simulink model "Lessons_Scheduled_Completed"  (R2024b)
settings: Solver=VariableStepAuto  StartTime=0.0  StopTime=365  RelTol=1e-3
undefined symbols (not defined in the file): m, n
settings Model: Creator=lerat  LastModifiedBy=lerat

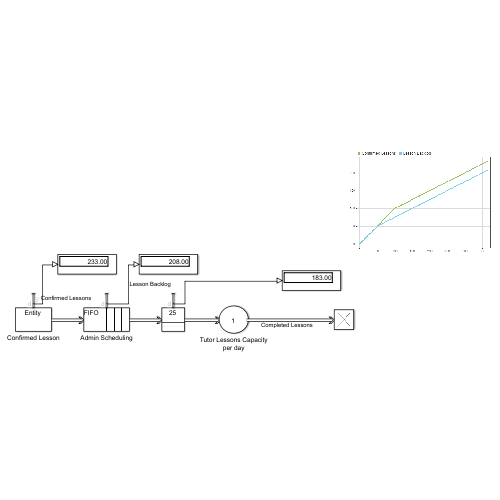
[thumbnail: Simulink's stored preview of the top-level diagram]
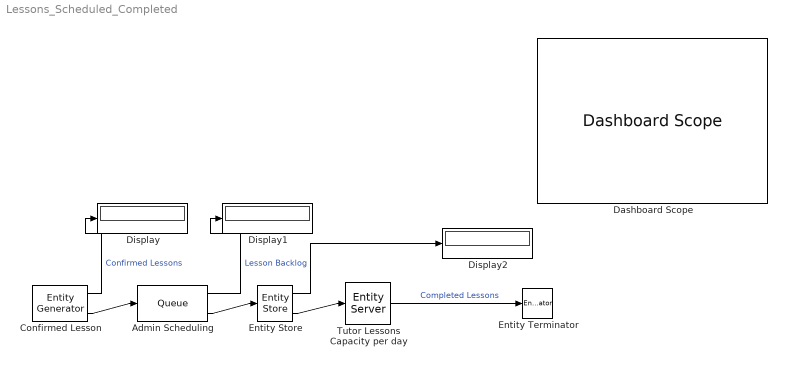
== system Lessons_Scheduled_Completed ==
  Admin Scheduling : Queue  InputPortMessageModes=m  OutputPortMessageModes=n,m  NumberEntitiesDeparted=on
      settings: OutputPortMap=o0,o5
  Confirmed Lesson : EntityGenerator  OutputPortMessageModes=n,m  NumberEntitiesDeparted=on  EntityType=Structured  EntityTypeName=Entity
      settings: OutputPortMap=o0,o3
  Dashboard Scope : DashboardScope
  Display : Display
      settings: Format=bank
  Display1 : Display
      settings: Format=bank
  Display2 : Display
      settings: Format=bank
  Entity Store : EntityStore  InputPortMessageModes=m  OutputPortMessageModes=n,m  NumberEntitiesDeparted=on
      settings: OutputPortMap=o0,o4
  Entity Terminator : EntityTerminator  InputPortMessageModes=m
  Tutor Lessons Capacity per day : EntityServer  InputPortMessageModes=m  OutputPortMessageModes=m  Capacity=1  ServiceTimeValue=2
  wires:
  Confirmed Lesson/2 -> Admin Scheduling/1
  Confirmed Lesson/1 -> Display/1  "Confirmed Lessons"
  Admin Scheduling/1 -> Display1/1  "Lesson Backlog"
  Admin Scheduling/2 -> Entity Store/1
  Tutor Lessons Capacity per day/1 -> Entity Terminator/1  "Completed Lessons"
  Entity Store/2 -> Tutor Lessons Capacity per day/1
  Entity Store/1 -> Display2/1
